simulink model "task20_8"  (R2021a)
settings: Solver=VariableStepAuto  StartTime=0.0  StopTime=10.0  RelTol=1e-3
settings Model: Creator=reemb  LastModifiedBy=reemb

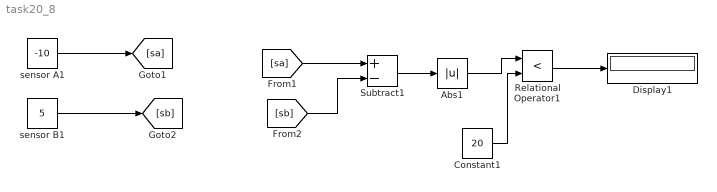
== system task20_8 ==
  Abs1 : Abs
  Constant1 : Constant  Value=20
  Display1 : Display
  Relational Operator1 : RelationalOperator  Operator=<  OutDataTypeStr=boolean  RndMeth=Simplest
  Subtract1 : Sum  Inputs=+-
  sensor A1 : Constant  Value=-10
  sensor B1 : Constant  Value=5
  wires:
  sensor A1/1 -> [sa]
  sensor B1/1 -> [sb]
  [sa] -> Subtract1/1
  [sb] -> Subtract1/2
  Constant1/1 -> Relational Operator1/2
  Abs1/1 -> Relational Operator1/1
  Relational Operator1/1 -> Display1/1
  Subtract1/1 -> Abs1/1
